simulink model "VSEModel"  (R2025b)
settings: Solver=VariableStepAuto  StartTime=0.0  StopTime=10.0  RelTol=1e-3
values from neighbouring files (symbols this model uses):
  K_TIRE_ROLLING_RADIUS = 0.3    [VSEModel.sldd]
  K_VSE_FILT_TC = 0.05    [VSEModel.sldd]
  K_VSE_MAX_SPEED = 300.0    [VSEModel.sldd]
settings Model: DataDictionary=VSEModel.sldd  Creator=farzanehtatari  LastModifiedBy=farzanehtatari

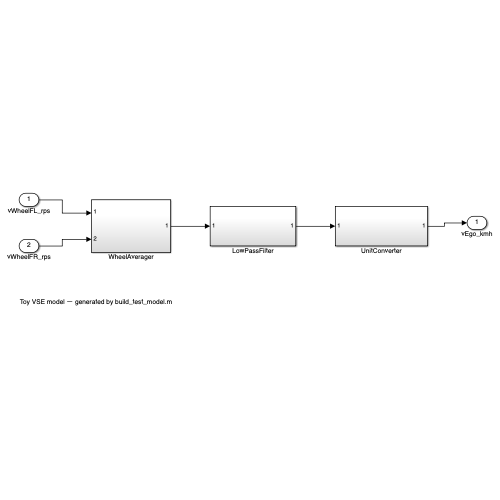
[thumbnail: Simulink's stored preview of the top-level diagram]
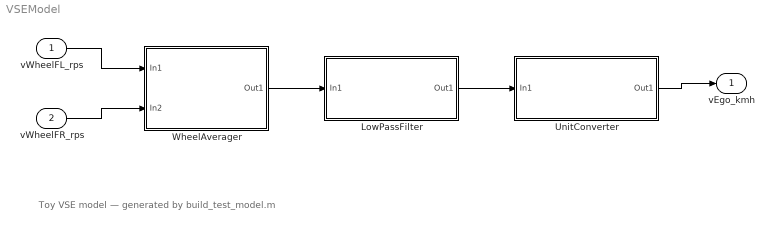
== system VSEModel ==
  note: Toy VSE model — generated by build_test_model.m
  vWheelFL_rps : Inport
  vWheelFR_rps : Inport  Port=2
  LowPassFilter : Subsystem
  UnitConverter : Subsystem
  WheelAverager : Subsystem
  vEgo_kmh : Outport
  wires:
  vWheelFL_rps/1 -> WheelAverager/1(In1)
  vWheelFR_rps/1 -> WheelAverager/2(In2)
  WheelAverager/1(Out1) -> LowPassFilter/1(In1)
  LowPassFilter/1(Out1) -> UnitConverter/1(In1)
  UnitConverter/1(Out1) -> vEgo_kmh/1

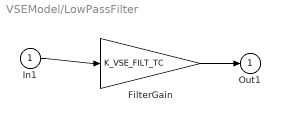
== system VSEModel/LowPassFilter ==
  In1 : Inport
  FilterGain : Gain  Gain=K_VSE_FILT_TC
  Out1 : Outport
  wires:
  In1/1 -> FilterGain/1
  FilterGain/1 -> Out1/1

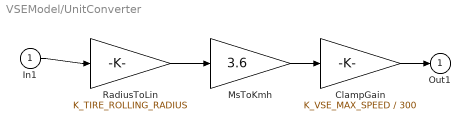
== system VSEModel/UnitConverter ==
  In1 : Inport
  ClampGain : Gain  Gain=K_VSE_MAX_SPEED / 300
  MsToKmh : Gain  Gain=3.6
  RadiusToLin : Gain  Gain=K_TIRE_ROLLING_RADIUS
  Out1 : Outport
  wires:
  In1/1 -> RadiusToLin/1
  RadiusToLin/1 -> MsToKmh/1
  MsToKmh/1 -> ClampGain/1
  ClampGain/1 -> Out1/1

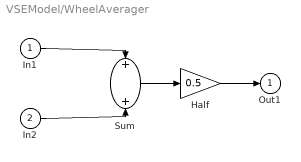
== system VSEModel/WheelAverager ==
  In1 : Inport
  In2 : Inport  Port=2
  Half : Gain  Gain=0.5
  Sum : Sum
  Out1 : Outport
  wires:
  In1/1 -> Sum/1
  In2/1 -> Sum/2
  Sum/1 -> Half/1
  Half/1 -> Out1/1
